simulink model "Factorial_WhileLoop"  (R2021a)
settings: Solver=VariableStepAuto  StartTime=0.0  StopTime=10.0  RelTol=1e-3
settings Model: Creator=NoteBook  LastModifiedBy=NoteBook

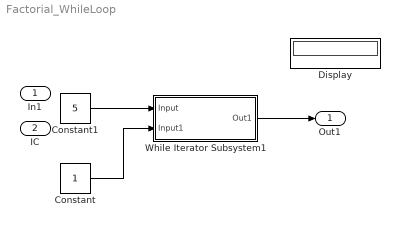
== system Factorial_WhileLoop ==
  In1 : Inport
  IC : Inport  Port=2
  Constant : Constant  OutDataTypeStr=uint8
  Constant1 : Constant  Value=5  OutDataTypeStr=uint8
  Display : Display
  While Iterator Subsystem1 : Subsystem  TreatAsAtomicUnit=on
  Out1 : Outport  OutDataTypeStr=uint32
  wires:
  While Iterator Subsystem1/1(Out1) -> Out1/1
  Constant1/1 -> While Iterator Subsystem1/1(Input)
  Constant/1 -> While Iterator Subsystem1/2(Input1)

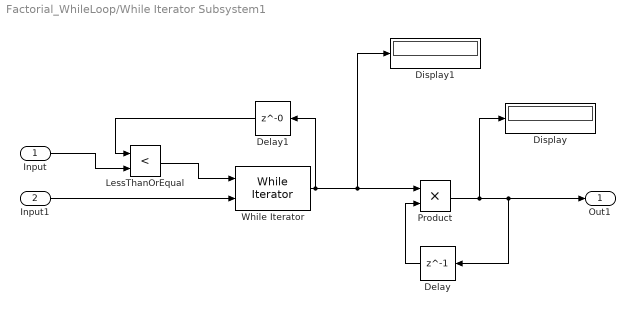
== system Factorial_WhileLoop/While Iterator Subsystem1 ==
  Input : Inport  OutDataTypeStr=uint8
  Input1 : Inport  Port=2  OutDataTypeStr=uint8
  Delay : Delay  DelayLength=1  InitialCondition=1
  Delay1 : Delay  DelayLength=0  InitialCondition=0
  Display : Display
  Display1 : Display
  LessThanOrEqual : RelationalOperator  Operator=<  OutDataTypeStr=boolean  RndMeth=Simplest
  Product : Product  OutDataTypeStr=uint32
  While Iterator : WhileIterator  MaxIters=-1  ShowIterationPort=on  OutputDataType=uint32
  Out1 : Outport  OutDataTypeStr=uint32
  wires:
  Input1/1 -> While Iterator/2
  While Iterator/1 -> Delay1/1, Display1/1, Product/1
  Product/1 -> Display/1, Out1/1, Delay/1
  Delay/1 -> Product/2
  Input/1 -> LessThanOrEqual/2
  Delay1/1 -> LessThanOrEqual/1
  LessThanOrEqual/1 -> While Iterator/1
